simulink model "parallel2ser"  (R2013b)
settings: Solver=FixedStepDiscrete  StartTime=0.0  StopTime=20  FixedStep=0.1  RelTol=1e-3
libraries: simulink x2
settings Model: Creator=mainster  LastModifiedBy=mainster

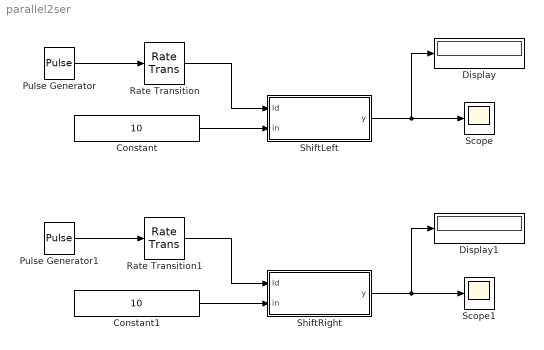
== system parallel2ser ==
  " ShiftLeft" : Subsystem  TreatAsAtomicUnit=on
  " ShiftRight" : Subsystem  TreatAsAtomicUnit=on
  Constant : Constant  Value=10  VectorParams1D=off  SampleTime=-1
      settings: SamplingMode=Frame based
  Constant1 : Constant  Value=10  VectorParams1D=off  SampleTime=-1
      settings: SamplingMode=Frame based
  Display : Display
      settings: Format=binary (Stored Integer)
  Display1 : Display
      settings: Format=binary (Stored Integer)
  Pulse Generator : DiscretePulseGenerator
  Pulse Generator1 : DiscretePulseGenerator
  Rate Transition : RateTransition  OutPortSampleTime=0.1
  Rate Transition1 : RateTransition  OutPortSampleTime=0.1
  Scope : Scope
      settings: ShowLegends=on  TimeRange=20
  Scope1 : Scope
      settings: ShowLegends=on  TimeRange=20
  wires:
  Constant/1 -> " ShiftLeft"/2(in)
  " ShiftLeft"/1(y) -> Display/1, Scope/1
  Pulse Generator/1 -> Rate Transition/1
  Rate Transition/1 -> " ShiftLeft"/1(ld)
  Constant1/1 -> " ShiftRight"/2(in)
  " ShiftRight"/1(y) -> Display1/1, Scope1/1
  Pulse Generator1/1 -> Rate Transition1/1
  Rate Transition1/1 -> " ShiftRight"/1(ld)

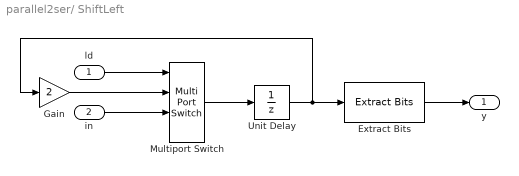
== system parallel2ser/ ShiftLeft ==
  ld : Inport
  in : Inport  Port=2
  Extract Bits : simulink/Logic and Bit Operations/Extract Bits  bitsToExtract=Range of bits  numBits=8  bitIdxRange=[15 15]  outScalingMode=Treat bit field as an integer
  Gain : Gain  Gain=2  ParamDataTypeStr=Inherit: Inherit from 'Gain'
  Multiport Switch : MultiPortSwitch  DataPortOrder=Zero-based contiguous  DiagnosticForDefault=Warning
  Unit Delay : UnitDelay  SampleTime=-1
  y : Outport
  wires:
  ld/1 -> Multiport Switch/1
  in/1 -> Multiport Switch/3
  Gain/1 -> Multiport Switch/2
  Multiport Switch/1 -> Unit Delay/1
  Unit Delay/1 -> Gain/1, Extract Bits/1
  Extract Bits/1 -> y/1

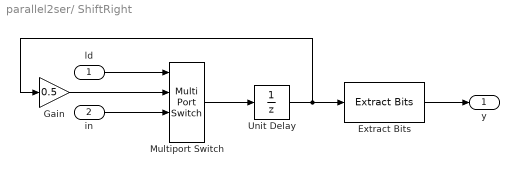
== system parallel2ser/ ShiftRight ==
  ld : Inport
  in : Inport  Port=2
  Extract Bits : simulink/Logic and Bit Operations/Extract Bits  bitsToExtract=Range of bits  numBits=8  bitIdxRange=[0 0]  outScalingMode=Treat bit field as an integer
  Gain : Gain  Gain=0.5  ParamDataTypeStr=Inherit: Inherit from 'Gain'
  Multiport Switch : MultiPortSwitch  DataPortOrder=Zero-based contiguous  DiagnosticForDefault=Warning
  Unit Delay : UnitDelay  SampleTime=-1
  y : Outport
  wires:
  ld/1 -> Multiport Switch/1
  in/1 -> Multiport Switch/3
  Gain/1 -> Multiport Switch/2
  Multiport Switch/1 -> Unit Delay/1
  Unit Delay/1 -> Gain/1, Extract Bits/1
  Extract Bits/1 -> y/1
